simulink model "IEEE34_SPSload"  (R2021b)
settings: Solver=ode4  StartTime=0.0  StopTime=5  FixedStep=50e-6  RelTol=1e-3
PreLoadFcn:
  | pGain = 0.05; % Gain of random perturbation (pu)
  | pGainAP = 0.01; % Gain of sinusoidal active power variation (pu)
  | pGainRP = 0.01; % Gain of sinusoidal reactive power variation (pu)
  | pFreqAP = 0.03; % Frequency of sinusoidal active power variation (Hz)
  | pFreqRP = 0.03; % Frequency of sinusoidal reactive power variation (Hz)
  | 
  | init_IEEE34nodetestfeeder;
InitFcn:
  | pGain = 0.05; % Gain of random perturbation (pu)
  | pGainAP = 0.01; % Gain of sinusoidal active power variation (pu)
  | pGainRP = 0.01; % Gain of sinusoidal reactive power variation (pu)
  | pFreqAP = 0.03; % Frequency of sinusoidal active power variation (Hz)
  | pFreqRP = 0.03; % Frequency of sinusoidal reactive power variation (Hz)
  | 
  | init_IEEE34nodetestfeeder;
values from neighbouring files (symbols this model uses):
  fNom = f    (= 60)    [init_IEEE34nodetestfeeder.m]
  loadcoeff = 1.0    (= 1)    [init_IEEE34nodetestfeeder.m]
  Ts = 50e-6    (= 5e-05)    [init_IEEE34nodetestfeeder.m]
  vNomMV = VsubL    (= 24900)    [init_IEEE34nodetestfeeder.m]
  VsubL = 24.9e3    (= 24900)    [init_IEEE34nodetestfeeder.m]
  VxfmL = 4.16e3    (= 4160)    [init_IEEE34nodetestfeeder.m]
undefined symbols (not defined in the file or in its folder): Ac, Bc, Cc, Dc, find_system, j
libraries: spsSeriesRLCBranchLib x418, spsGroundLib x242, simulink_extras x176, spsVoltageMeasurementLib x106, spsRMSLib x96, spsControlledCurrentSourceLib x94, spsThreePhaseVIMeasurementLib x37, spsMutualInductanceLib x24, spsCurrentMeasurementLib x12, spsOnDelayLib x12, spsLinearTransformerLib x6, spsControlledVoltageSourceLib x6
(part 9 of 33)

== system IEEE34_SPSload/SM_IEEE34/DL_802-1/Load B ==
  Controlled Current Source : spsControlledCurrentSourceLib/Controlled Current Source  Initialize=on  Source_Type=AC  Amplitude=0  Phase=0  Frequency=0  Measurements=None
  Gain : Gain  Gain=-1
  Measurement list : Subsystem
  PQ : Ground
  Series RLC Branch : spsSeriesRLCBranchLib/Series RLC Branch  LConnTagsString=__new0  RConnTagsString=__new0  BranchType=R  Resistance=1e8  Inductance=1e-3  SetiL0=off  InitialCurrent=0  Capacitance=1e-6  Setx0=off  InitialVoltage=0  Measurements=None
  Voltage Measurement1 : spsVoltageMeasurementLib/Voltage Measurement  PhasorSimulation=off  OutputType=Complex  PSBequivalent=0
  model : Subsystem
  a : PMIOPort  Tag=PMCPort  Side=Left
  b : PMIOPort  Tag=PMCPort  Port=2  Side=Left
  m : Outport  InitialOutput=[0,0,0]  VectorParamsAs1DForOutWhenUnconnected=off
  wires:
  Gain/1 -> Controlled Current Source/1
  Measurement list/1(Out1) -> m/1
  model/1(i) -> Gain/1
  Voltage Measurement1/1 -> model/1(v)
  PQ/1 -> model/2(PQ)
  model/2(m) -> Measurement list/1(In1)
  connections:
  Series RLC Branch/RConn1 -- Voltage Measurement1/LConn2 -- b/RConn1 -- Controlled Current Source/LConn1
  a/RConn1 -- Series RLC Branch/LConn1 -- Controlled Current Source/RConn1 -- Voltage Measurement1/LConn1

== system IEEE34_SPSload/SM_IEEE34/DL_802-1/Load B1 ==
  Controlled Current Source : spsControlledCurrentSourceLib/Controlled Current Source  Initialize=on  Source_Type=AC  Amplitude=0  Phase=0  Frequency=0  Measurements=None
  Gain : Gain  Gain=-1
  Measurement list : Subsystem
  PQ : Ground
  Series RLC Branch : spsSeriesRLCBranchLib/Series RLC Branch  LConnTagsString=__new0  RConnTagsString=__new0  BranchType=R  Resistance=1e8  Inductance=1e-3  SetiL0=off  InitialCurrent=0  Capacitance=1e-6  Setx0=off  InitialVoltage=0  Measurements=None
  Voltage Measurement1 : spsVoltageMeasurementLib/Voltage Measurement  PhasorSimulation=off  OutputType=Complex  PSBequivalent=0
  model : Subsystem
  a : PMIOPort  Tag=PMCPort  Side=Left
  b : PMIOPort  Tag=PMCPort  Port=2  Side=Left
  m : Outport  InitialOutput=[0,0,0]  VectorParamsAs1DForOutWhenUnconnected=off
  wires:
  model/2(m) -> Measurement list/1(In1)
  PQ/1 -> model/2(PQ)
  Voltage Measurement1/1 -> model/1(v)
  model/1(i) -> Gain/1
  Measurement list/1(Out1) -> m/1
  Gain/1 -> Controlled Current Source/1
  connections:
  Voltage Measurement1/LConn1 -- Controlled Current Source/RConn1 -- Series RLC Branch/LConn1 -- a/RConn1
  Controlled Current Source/LConn1 -- b/RConn1 -- Voltage Measurement1/LConn2 -- Series RLC Branch/RConn1

== system IEEE34_SPSload/SM_IEEE34/DL_802-1/Load C ==
  Controlled Current Source : spsControlledCurrentSourceLib/Controlled Current Source  Initialize=on  Source_Type=AC  Amplitude=0  Phase=0  Frequency=0  Measurements=None
  Gain : Gain  Gain=-1
  Measurement list : Subsystem
  PQ : Ground
  Series RLC Branch : spsSeriesRLCBranchLib/Series RLC Branch  LConnTagsString=__new0  RConnTagsString=__new0  BranchType=R  Resistance=1e8  Inductance=1e-3  SetiL0=off  InitialCurrent=0  Capacitance=1e-6  Setx0=off  InitialVoltage=0  Measurements=None
  Voltage Measurement1 : spsVoltageMeasurementLib/Voltage Measurement  PhasorSimulation=off  OutputType=Complex  PSBequivalent=0
  model : Subsystem
  a : PMIOPort  Tag=PMCPort  Side=Left
  b : PMIOPort  Tag=PMCPort  Port=2  Side=Left
  m : Outport  InitialOutput=[0,0,0]  VectorParamsAs1DForOutWhenUnconnected=off
  wires:
  model/2(m) -> Measurement list/1(In1)
  PQ/1 -> model/2(PQ)
  Voltage Measurement1/1 -> model/1(v)
  model/1(i) -> Gain/1
  Measurement list/1(Out1) -> m/1
  Gain/1 -> Controlled Current Source/1
  connections:
  Voltage Measurement1/LConn1 -- a/RConn1 -- Series RLC Branch/LConn1 -- Controlled Current Source/RConn1
  Voltage Measurement1/LConn2 -- b/RConn1 -- Series RLC Branch/RConn1 -- Controlled Current Source/LConn1

== system IEEE34_SPSload/SM_IEEE34/DL_802-2/Load B ==
  Controlled Current Source : spsControlledCurrentSourceLib/Controlled Current Source  Initialize=on  Source_Type=AC  Amplitude=0  Phase=0  Frequency=0  Measurements=None
  Gain : Gain  Gain=-1
  Measurement list : Subsystem
  PQ : Ground
  Series RLC Branch : spsSeriesRLCBranchLib/Series RLC Branch  LConnTagsString=__new0  RConnTagsString=__new0  BranchType=R  Resistance=1e8  Inductance=1e-3  SetiL0=off  InitialCurrent=0  Capacitance=1e-6  Setx0=off  InitialVoltage=0  Measurements=None
  Voltage Measurement1 : spsVoltageMeasurementLib/Voltage Measurement  PhasorSimulation=off  OutputType=Complex  PSBequivalent=0
  model : Subsystem
  a : PMIOPort  Tag=PMCPort  Side=Left
  b : PMIOPort  Tag=PMCPort  Port=2  Side=Left
  m : Outport  InitialOutput=[0,0,0]  VectorParamsAs1DForOutWhenUnconnected=off
  wires:
  model/2(m) -> Measurement list/1(In1)
  PQ/1 -> model/2(PQ)
  Voltage Measurement1/1 -> model/1(v)
  model/1(i) -> Gain/1
  Measurement list/1(Out1) -> m/1
  Gain/1 -> Controlled Current Source/1
  connections:
  Voltage Measurement1/LConn1 -- Controlled Current Source/RConn1 -- Series RLC Branch/LConn1 -- a/RConn1
  Controlled Current Source/LConn1 -- b/RConn1 -- Voltage Measurement1/LConn2 -- Series RLC Branch/RConn1

== system IEEE34_SPSload/SM_IEEE34/DL_802-2/Load B1 ==
  Controlled Current Source : spsControlledCurrentSourceLib/Controlled Current Source  Initialize=on  Source_Type=AC  Amplitude=0  Phase=0  Frequency=0  Measurements=None
  Gain : Gain  Gain=-1
  Measurement list : Subsystem
  PQ : Ground
  Series RLC Branch : spsSeriesRLCBranchLib/Series RLC Branch  LConnTagsString=__new0  RConnTagsString=__new0  BranchType=R  Resistance=1e8  Inductance=1e-3  SetiL0=off  InitialCurrent=0  Capacitance=1e-6  Setx0=off  InitialVoltage=0  Measurements=None
  Voltage Measurement1 : spsVoltageMeasurementLib/Voltage Measurement  PhasorSimulation=off  OutputType=Complex  PSBequivalent=0
  model : Subsystem
  a : PMIOPort  Tag=PMCPort  Side=Left
  b : PMIOPort  Tag=PMCPort  Port=2  Side=Left
  m : Outport  InitialOutput=[0,0,0]  VectorParamsAs1DForOutWhenUnconnected=off
  wires:
  Gain/1 -> Controlled Current Source/1
  Measurement list/1(Out1) -> m/1
  model/1(i) -> Gain/1
  Voltage Measurement1/1 -> model/1(v)
  PQ/1 -> model/2(PQ)
  model/2(m) -> Measurement list/1(In1)
  connections:
  Series RLC Branch/RConn1 -- Voltage Measurement1/LConn2 -- b/RConn1 -- Controlled Current Source/LConn1
  a/RConn1 -- Series RLC Branch/LConn1 -- Controlled Current Source/RConn1 -- Voltage Measurement1/LConn1

== system IEEE34_SPSload/SM_IEEE34/DL_802-2/Load C ==
  Controlled Current Source : spsControlledCurrentSourceLib/Controlled Current Source  Initialize=on  Source_Type=AC  Amplitude=0  Phase=0  Frequency=0  Measurements=None
  Gain : Gain  Gain=-1
  Measurement list : Subsystem
  PQ : Ground
  Series RLC Branch : spsSeriesRLCBranchLib/Series RLC Branch  LConnTagsString=__new0  RConnTagsString=__new0  BranchType=R  Resistance=1e8  Inductance=1e-3  SetiL0=off  InitialCurrent=0  Capacitance=1e-6  Setx0=off  InitialVoltage=0  Measurements=None
  Voltage Measurement1 : spsVoltageMeasurementLib/Voltage Measurement  PhasorSimulation=off  OutputType=Complex  PSBequivalent=0
  model : Subsystem
  a : PMIOPort  Tag=PMCPort  Side=Left
  b : PMIOPort  Tag=PMCPort  Port=2  Side=Left
  m : Outport  InitialOutput=[0,0,0]  VectorParamsAs1DForOutWhenUnconnected=off
  wires:
  Gain/1 -> Controlled Current Source/1
  Measurement list/1(Out1) -> m/1
  model/1(i) -> Gain/1
  Voltage Measurement1/1 -> model/1(v)
  PQ/1 -> model/2(PQ)
  model/2(m) -> Measurement list/1(In1)
  connections:
  Controlled Current Source/LConn1 -- Series RLC Branch/RConn1 -- b/RConn1 -- Voltage Measurement1/LConn2
  Controlled Current Source/RConn1 -- Series RLC Branch/LConn1 -- a/RConn1 -- Voltage Measurement1/LConn1

== system IEEE34_SPSload/SM_IEEE34/DL_808-1/Load B ==
  Controlled Current Source : spsControlledCurrentSourceLib/Controlled Current Source  Initialize=on  Source_Type=AC  Amplitude=0  Phase=0  Frequency=0  Measurements=None
  Gain : Gain  Gain=-1
  Measurement list : Subsystem
  PQ : Ground
  Series RLC Branch : spsSeriesRLCBranchLib/Series RLC Branch  LConnTagsString=__new0  RConnTagsString=__new0  BranchType=R  Resistance=1e8  Inductance=1e-3  SetiL0=off  InitialCurrent=0  Capacitance=1e-6  Setx0=off  InitialVoltage=0  Measurements=None
  Voltage Measurement1 : spsVoltageMeasurementLib/Voltage Measurement  PhasorSimulation=off  OutputType=Complex  PSBequivalent=0
  model : Subsystem
  a : PMIOPort  Tag=PMCPort  Side=Left
  b : PMIOPort  Tag=PMCPort  Port=2  Side=Left
  m : Outport  InitialOutput=[0,0,0]  VectorParamsAs1DForOutWhenUnconnected=off
  wires:
  Gain/1 -> Controlled Current Source/1
  Measurement list/1(Out1) -> m/1
  model/1(i) -> Gain/1
  Voltage Measurement1/1 -> model/1(v)
  PQ/1 -> model/2(PQ)
  model/2(m) -> Measurement list/1(In1)
  connections:
  Controlled Current Source/LConn1 -- b/RConn1 -- Series RLC Branch/RConn1 -- Voltage Measurement1/LConn2
  Controlled Current Source/RConn1 -- a/RConn1 -- Series RLC Branch/LConn1 -- Voltage Measurement1/LConn1

== system IEEE34_SPSload/SM_IEEE34/DL_808-810/Load B ==
  Controlled Current Source : spsControlledCurrentSourceLib/Controlled Current Source  Initialize=on  Source_Type=AC  Amplitude=0  Phase=0  Frequency=0  Measurements=None
  Gain : Gain  Gain=-1
  Measurement list : Subsystem
  PQ : Ground
  Series RLC Branch : spsSeriesRLCBranchLib/Series RLC Branch  LConnTagsString=__new0  RConnTagsString=__new0  BranchType=R  Resistance=1e8  Inductance=1e-3  SetiL0=off  InitialCurrent=0  Capacitance=1e-6  Setx0=off  InitialVoltage=0  Measurements=None
  Voltage Measurement1 : spsVoltageMeasurementLib/Voltage Measurement  PhasorSimulation=off  OutputType=Complex  PSBequivalent=0
  model : Subsystem
  a : PMIOPort  Tag=PMCPort  Side=Left
  b : PMIOPort  Tag=PMCPort  Port=2  Side=Left
  m : Outport  InitialOutput=[0,0,0]  VectorParamsAs1DForOutWhenUnconnected=off
  wires:
  model/2(m) -> Measurement list/1(In1)
  PQ/1 -> model/2(PQ)
  Voltage Measurement1/1 -> model/1(v)
  model/1(i) -> Gain/1
  Measurement list/1(Out1) -> m/1
  Gain/1 -> Controlled Current Source/1
  connections:
  Voltage Measurement1/LConn1 -- Series RLC Branch/LConn1 -- a/RConn1 -- Controlled Current Source/RConn1
  Voltage Measurement1/LConn2 -- Series RLC Branch/RConn1 -- b/RConn1 -- Controlled Current Source/LConn1

== system IEEE34_SPSload/SM_IEEE34/DL_816-1/Load B ==
  Controlled Current Source : spsControlledCurrentSourceLib/Controlled Current Source  Initialize=on  Source_Type=AC  Amplitude=0  Phase=0  Frequency=0  Measurements=None
  Gain : Gain  Gain=-1
  Measurement list : Subsystem
  PQ : Ground
  Series RLC Branch : spsSeriesRLCBranchLib/Series RLC Branch  LConnTagsString=__new0  RConnTagsString=__new0  BranchType=R  Resistance=1e8  Inductance=1e-3  SetiL0=off  InitialCurrent=0  Capacitance=1e-6  Setx0=off  InitialVoltage=0  Measurements=None
  Voltage Measurement1 : spsVoltageMeasurementLib/Voltage Measurement  PhasorSimulation=off  OutputType=Complex  PSBequivalent=0
  model : Subsystem
  a : PMIOPort  Tag=PMCPort  Side=Left
  b : PMIOPort  Tag=PMCPort  Port=2  Side=Left
  m : Outport  InitialOutput=[0,0,0]  VectorParamsAs1DForOutWhenUnconnected=off
  wires:
  Gain/1 -> Controlled Current Source/1
  Measurement list/1(Out1) -> m/1
  model/1(i) -> Gain/1
  Voltage Measurement1/1 -> model/1(v)
  PQ/1 -> model/2(PQ)
  model/2(m) -> Measurement list/1(In1)
  connections:
  Controlled Current Source/LConn1 -- b/RConn1 -- Series RLC Branch/RConn1 -- Voltage Measurement1/LConn2
  Controlled Current Source/RConn1 -- a/RConn1 -- Series RLC Branch/LConn1 -- Voltage Measurement1/LConn1

== system IEEE34_SPSload/SM_IEEE34/DL_816-1/Load B1 ==
  Controlled Current Source : spsControlledCurrentSourceLib/Controlled Current Source  Initialize=on  Source_Type=AC  Amplitude=0  Phase=0  Frequency=0  Measurements=None
  Gain : Gain  Gain=-1
  Measurement list : Subsystem
  PQ : Ground
  Series RLC Branch : spsSeriesRLCBranchLib/Series RLC Branch  LConnTagsString=__new0  RConnTagsString=__new0  BranchType=R  Resistance=1e8  Inductance=1e-3  SetiL0=off  InitialCurrent=0  Capacitance=1e-6  Setx0=off  InitialVoltage=0  Measurements=None
  Voltage Measurement1 : spsVoltageMeasurementLib/Voltage Measurement  PhasorSimulation=off  OutputType=Complex  PSBequivalent=0
  model : Subsystem
  a : PMIOPort  Tag=PMCPort  Side=Left
  b : PMIOPort  Tag=PMCPort  Port=2  Side=Left
  m : Outport  InitialOutput=[0,0,0]  VectorParamsAs1DForOutWhenUnconnected=off
  wires:
  model/2(m) -> Measurement list/1(In1)
  PQ/1 -> model/2(PQ)
  Voltage Measurement1/1 -> model/1(v)
  model/1(i) -> Gain/1
  Measurement list/1(Out1) -> m/1
  Gain/1 -> Controlled Current Source/1
  connections:
  Voltage Measurement1/LConn1 -- Series RLC Branch/LConn1 -- a/RConn1 -- Controlled Current Source/RConn1
  Voltage Measurement1/LConn2 -- Series RLC Branch/RConn1 -- b/RConn1 -- Controlled Current Source/LConn1

== system IEEE34_SPSload/SM_IEEE34/DL_816-1/Load B2 ==
  Controlled Current Source : spsControlledCurrentSourceLib/Controlled Current Source  Initialize=on  Source_Type=AC  Amplitude=0  Phase=0  Frequency=0  Measurements=None
  Gain : Gain  Gain=-1
  Measurement list : Subsystem
  PQ : Ground
  Series RLC Branch : spsSeriesRLCBranchLib/Series RLC Branch  LConnTagsString=__new0  RConnTagsString=__new0  BranchType=R  Resistance=1e8  Inductance=1e-3  SetiL0=off  InitialCurrent=0  Capacitance=1e-6  Setx0=off  InitialVoltage=0  Measurements=None
  Voltage Measurement1 : spsVoltageMeasurementLib/Voltage Measurement  PhasorSimulation=off  OutputType=Complex  PSBequivalent=0
  model : Subsystem
  a : PMIOPort  Tag=PMCPort  Side=Left
  b : PMIOPort  Tag=PMCPort  Port=2  Side=Left
  m : Outport  InitialOutput=[0,0,0]  VectorParamsAs1DForOutWhenUnconnected=off
  wires:
  model/2(m) -> Measurement list/1(In1)
  PQ/1 -> model/2(PQ)
  Voltage Measurement1/1 -> model/1(v)
  model/1(i) -> Gain/1
  Measurement list/1(Out1) -> m/1
  Gain/1 -> Controlled Current Source/1
  connections:
  Voltage Measurement1/LConn1 -- Series RLC Branch/LConn1 -- a/RConn1 -- Controlled Current Source/RConn1
  Voltage Measurement1/LConn2 -- Series RLC Branch/RConn1 -- b/RConn1 -- Controlled Current Source/LConn1

== system IEEE34_SPSload/SM_IEEE34/DL_816-824/Load B ==
  Controlled Current Source : spsControlledCurrentSourceLib/Controlled Current Source  Initialize=on  Source_Type=AC  Amplitude=0  Phase=0  Frequency=0  Measurements=None
  Gain : Gain  Gain=-1
  Measurement list : Subsystem
  PQ : Ground
  Series RLC Branch : spsSeriesRLCBranchLib/Series RLC Branch  LConnTagsString=__new0  RConnTagsString=__new0  BranchType=R  Resistance=1e8  Inductance=1e-3  SetiL0=off  InitialCurrent=0  Capacitance=1e-6  Setx0=off  InitialVoltage=0  Measurements=None
  Voltage Measurement1 : spsVoltageMeasurementLib/Voltage Measurement  PhasorSimulation=off  OutputType=Complex  PSBequivalent=0
  model : Subsystem
  a : PMIOPort  Tag=PMCPort  Side=Left
  b : PMIOPort  Tag=PMCPort  Port=2  Side=Left
  m : Outport  InitialOutput=[0,0,0]  VectorParamsAs1DForOutWhenUnconnected=off
  wires:
  model/2(m) -> Measurement list/1(In1)
  PQ/1 -> model/2(PQ)
  Voltage Measurement1/1 -> model/1(v)
  model/1(i) -> Gain/1
  Measurement list/1(Out1) -> m/1
  Gain/1 -> Controlled Current Source/1
  connections:
  Voltage Measurement1/LConn1 -- Series RLC Branch/LConn1 -- a/RConn1 -- Controlled Current Source/RConn1
  Voltage Measurement1/LConn2 -- Series RLC Branch/RConn1 -- b/RConn1 -- Controlled Current Source/LConn1

== system IEEE34_SPSload/SM_IEEE34/DL_816-824/Load B1 ==
  Controlled Current Source : spsControlledCurrentSourceLib/Controlled Current Source  Initialize=on  Source_Type=AC  Amplitude=0  Phase=0  Frequency=0  Measurements=None
  Gain : Gain  Gain=-1
  Measurement list : Subsystem
  PQ : Ground
  Series RLC Branch : spsSeriesRLCBranchLib/Series RLC Branch  LConnTagsString=__new0  RConnTagsString=__new0  BranchType=R  Resistance=1e8  Inductance=1e-3  SetiL0=off  InitialCurrent=0  Capacitance=1e-6  Setx0=off  InitialVoltage=0  Measurements=None
  Voltage Measurement1 : spsVoltageMeasurementLib/Voltage Measurement  PhasorSimulation=off  OutputType=Complex  PSBequivalent=0
  model : Subsystem
  a : PMIOPort  Tag=PMCPort  Side=Left
  b : PMIOPort  Tag=PMCPort  Port=2  Side=Left
  m : Outport  InitialOutput=[0,0,0]  VectorParamsAs1DForOutWhenUnconnected=off
  wires:
  Gain/1 -> Controlled Current Source/1
  Measurement list/1(Out1) -> m/1
  model/1(i) -> Gain/1
  Voltage Measurement1/1 -> model/1(v)
  PQ/1 -> model/2(PQ)
  model/2(m) -> Measurement list/1(In1)
  connections:
  Controlled Current Source/LConn1 -- b/RConn1 -- Series RLC Branch/RConn1 -- Voltage Measurement1/LConn2
  Controlled Current Source/RConn1 -- a/RConn1 -- Series RLC Branch/LConn1 -- Voltage Measurement1/LConn1

== system IEEE34_SPSload/SM_IEEE34/DL_816-824/Load B2 ==
  Controlled Current Source : spsControlledCurrentSourceLib/Controlled Current Source  Initialize=on  Source_Type=AC  Amplitude=0  Phase=0  Frequency=0  Measurements=None
  Gain : Gain  Gain=-1
  Measurement list : Subsystem
  PQ : Ground
  Series RLC Branch : spsSeriesRLCBranchLib/Series RLC Branch  LConnTagsString=__new0  RConnTagsString=__new0  BranchType=R  Resistance=1e8  Inductance=1e-3  SetiL0=off  InitialCurrent=0  Capacitance=1e-6  Setx0=off  InitialVoltage=0  Measurements=None
  Voltage Measurement1 : spsVoltageMeasurementLib/Voltage Measurement  PhasorSimulation=off  OutputType=Complex  PSBequivalent=0
  model : Subsystem
  a : PMIOPort  Tag=PMCPort  Side=Left
  b : PMIOPort  Tag=PMCPort  Port=2  Side=Left
  m : Outport  InitialOutput=[0,0,0]  VectorParamsAs1DForOutWhenUnconnected=off
  wires:
  Gain/1 -> Controlled Current Source/1
  Measurement list/1(Out1) -> m/1
  model/1(i) -> Gain/1
  Voltage Measurement1/1 -> model/1(v)
  PQ/1 -> model/2(PQ)
  model/2(m) -> Measurement list/1(In1)
  connections:
  Controlled Current Source/LConn1 -- b/RConn1 -- Series RLC Branch/RConn1 -- Voltage Measurement1/LConn2
  Controlled Current Source/RConn1 -- a/RConn1 -- Series RLC Branch/LConn1 -- Voltage Measurement1/LConn1

== system IEEE34_SPSload/SM_IEEE34/DL_818-1/Load B ==
  Controlled Current Source : spsControlledCurrentSourceLib/Controlled Current Source  Initialize=on  Source_Type=AC  Amplitude=0  Phase=0  Frequency=0  Measurements=None
  Gain : Gain  Gain=-1
  Measurement list : Subsystem
  PQ : Ground
  Series RLC Branch : spsSeriesRLCBranchLib/Series RLC Branch  LConnTagsString=__new0  RConnTagsString=__new0  BranchType=R  Resistance=1e8  Inductance=1e-3  SetiL0=off  InitialCurrent=0  Capacitance=1e-6  Setx0=off  InitialVoltage=0  Measurements=None
  Voltage Measurement1 : spsVoltageMeasurementLib/Voltage Measurement  PhasorSimulation=off  OutputType=Complex  PSBequivalent=0
  model : Subsystem
  a : PMIOPort  Tag=PMCPort  Side=Left
  b : PMIOPort  Tag=PMCPort  Port=2  Side=Left
  m : Outport  InitialOutput=[0,0,0]  VectorParamsAs1DForOutWhenUnconnected=off
  wires:
  Gain/1 -> Controlled Current Source/1
  Measurement list/1(Out1) -> m/1
  model/1(i) -> Gain/1
  Voltage Measurement1/1 -> model/1(v)
  PQ/1 -> model/2(PQ)
  model/2(m) -> Measurement list/1(In1)
  connections:
  Controlled Current Source/LConn1 -- b/RConn1 -- Series RLC Branch/RConn1 -- Voltage Measurement1/LConn2
  Controlled Current Source/RConn1 -- a/RConn1 -- Series RLC Branch/LConn1 -- Voltage Measurement1/LConn1

== system IEEE34_SPSload/SM_IEEE34/DL_818-820/Load B ==
  Controlled Current Source : spsControlledCurrentSourceLib/Controlled Current Source  Initialize=on  Source_Type=AC  Amplitude=0  Phase=0  Frequency=0  Measurements=None
  Gain : Gain  Gain=-1
  Measurement list : Subsystem
  PQ : Ground
  Series RLC Branch : spsSeriesRLCBranchLib/Series RLC Branch  LConnTagsString=__new0  RConnTagsString=__new0  BranchType=R  Resistance=1e8  Inductance=1e-3  SetiL0=off  InitialCurrent=0  Capacitance=1e-6  Setx0=off  InitialVoltage=0  Measurements=None
  Voltage Measurement1 : spsVoltageMeasurementLib/Voltage Measurement  PhasorSimulation=off  OutputType=Complex  PSBequivalent=0
  model : Subsystem
  a : PMIOPort  Tag=PMCPort  Side=Left
  b : PMIOPort  Tag=PMCPort  Port=2  Side=Left
  m : Outport  InitialOutput=[0,0,0]  VectorParamsAs1DForOutWhenUnconnected=off
  wires:
  model/2(m) -> Measurement list/1(In1)
  PQ/1 -> model/2(PQ)
  Voltage Measurement1/1 -> model/1(v)
  model/1(i) -> Gain/1
  Measurement list/1(Out1) -> m/1
  Gain/1 -> Controlled Current Source/1
  connections:
  Voltage Measurement1/LConn1 -- Series RLC Branch/LConn1 -- a/RConn1 -- Controlled Current Source/RConn1
  Voltage Measurement1/LConn2 -- Series RLC Branch/RConn1 -- b/RConn1 -- Controlled Current Source/LConn1

== system IEEE34_SPSload/SM_IEEE34/DL_820-1/Load B ==
  Controlled Current Source : spsControlledCurrentSourceLib/Controlled Current Source  Initialize=on  Source_Type=AC  Amplitude=0  Phase=0  Frequency=0  Measurements=None
  Gain : Gain  Gain=-1
  Measurement list : Subsystem
  PQ : Ground
  Series RLC Branch : spsSeriesRLCBranchLib/Series RLC Branch  LConnTagsString=__new0  RConnTagsString=__new0  BranchType=R  Resistance=1e8  Inductance=1e-3  SetiL0=off  InitialCurrent=0  Capacitance=1e-6  Setx0=off  InitialVoltage=0  Measurements=None
  Voltage Measurement1 : spsVoltageMeasurementLib/Voltage Measurement  PhasorSimulation=off  OutputType=Complex  PSBequivalent=0
  model : Subsystem
  a : PMIOPort  Tag=PMCPort  Side=Left
  b : PMIOPort  Tag=PMCPort  Port=2  Side=Left
  m : Outport  InitialOutput=[0,0,0]  VectorParamsAs1DForOutWhenUnconnected=off
  wires:
  Gain/1 -> Controlled Current Source/1
  Measurement list/1(Out1) -> m/1
  model/1(i) -> Gain/1
  Voltage Measurement1/1 -> model/1(v)
  PQ/1 -> model/2(PQ)
  model/2(m) -> Measurement list/1(In1)
  connections:
  Controlled Current Source/LConn1 -- b/RConn1 -- Series RLC Branch/RConn1 -- Voltage Measurement1/LConn2
  Controlled Current Source/RConn1 -- a/RConn1 -- Series RLC Branch/LConn1 -- Voltage Measurement1/LConn1

== system IEEE34_SPSload/SM_IEEE34/DL_820-822/Load B ==
  Controlled Current Source : spsControlledCurrentSourceLib/Controlled Current Source  Initialize=on  Source_Type=AC  Amplitude=0  Phase=0  Frequency=0  Measurements=None
  Gain : Gain  Gain=-1
  Measurement list : Subsystem
  PQ : Ground
  Series RLC Branch : spsSeriesRLCBranchLib/Series RLC Branch  LConnTagsString=__new0  RConnTagsString=__new0  BranchType=R  Resistance=1e8  Inductance=1e-3  SetiL0=off  InitialCurrent=0  Capacitance=1e-6  Setx0=off  InitialVoltage=0  Measurements=None
  Voltage Measurement1 : spsVoltageMeasurementLib/Voltage Measurement  PhasorSimulation=off  OutputType=Complex  PSBequivalent=0
  model : Subsystem
  a : PMIOPort  Tag=PMCPort  Side=Left
  b : PMIOPort  Tag=PMCPort  Port=2  Side=Left
  m : Outport  InitialOutput=[0,0,0]  VectorParamsAs1DForOutWhenUnconnected=off
  wires:
  model/2(m) -> Measurement list/1(In1)
  PQ/1 -> model/2(PQ)
  Voltage Measurement1/1 -> model/1(v)
  model/1(i) -> Gain/1
  Measurement list/1(Out1) -> m/1
  Gain/1 -> Controlled Current Source/1
  connections:
  Voltage Measurement1/LConn1 -- Series RLC Branch/LConn1 -- a/RConn1 -- Controlled Current Source/RConn1
  Voltage Measurement1/LConn2 -- Series RLC Branch/RConn1 -- b/RConn1 -- Controlled Current Source/LConn1

== system IEEE34_SPSload/SM_IEEE34/DL_824-1/Load B ==
  Controlled Current Source : spsControlledCurrentSourceLib/Controlled Current Source  Initialize=on  Source_Type=AC  Amplitude=0  Phase=0  Frequency=0  Measurements=None
  Gain : Gain  Gain=-1
  Measurement list : Subsystem
  PQ : Ground
  Series RLC Branch : spsSeriesRLCBranchLib/Series RLC Branch  LConnTagsString=__new0  RConnTagsString=__new0  BranchType=R  Resistance=1e8  Inductance=1e-3  SetiL0=off  InitialCurrent=0  Capacitance=1e-6  Setx0=off  InitialVoltage=0  Measurements=None
  Voltage Measurement1 : spsVoltageMeasurementLib/Voltage Measurement  PhasorSimulation=off  OutputType=Complex  PSBequivalent=0
  model : Subsystem
  a : PMIOPort  Tag=PMCPort  Side=Left
  b : PMIOPort  Tag=PMCPort  Port=2  Side=Left
  m : Outport  InitialOutput=[0,0,0]  VectorParamsAs1DForOutWhenUnconnected=off
  wires:
  model/2(m) -> Measurement list/1(In1)
  PQ/1 -> model/2(PQ)
  Voltage Measurement1/1 -> model/1(v)
  model/1(i) -> Gain/1
  Measurement list/1(Out1) -> m/1
  Gain/1 -> Controlled Current Source/1
  connections:
  Voltage Measurement1/LConn1 -- Series RLC Branch/LConn1 -- a/RConn1 -- Controlled Current Source/RConn1
  Voltage Measurement1/LConn2 -- Series RLC Branch/RConn1 -- b/RConn1 -- Controlled Current Source/LConn1

== system IEEE34_SPSload/SM_IEEE34/DL_824-2/Load B ==
  Controlled Current Source : spsControlledCurrentSourceLib/Controlled Current Source  Initialize=on  Source_Type=AC  Amplitude=0  Phase=0  Frequency=0  Measurements=None
  Gain : Gain  Gain=-1
  Measurement list : Subsystem
  PQ : Ground
  Series RLC Branch : spsSeriesRLCBranchLib/Series RLC Branch  LConnTagsString=__new0  RConnTagsString=__new0  BranchType=R  Resistance=1e8  Inductance=1e-3  SetiL0=off  InitialCurrent=0  Capacitance=1e-6  Setx0=off  InitialVoltage=0  Measurements=None
  Voltage Measurement1 : spsVoltageMeasurementLib/Voltage Measurement  PhasorSimulation=off  OutputType=Complex  PSBequivalent=0
  model : Subsystem
  a : PMIOPort  Tag=PMCPort  Side=Left
  b : PMIOPort  Tag=PMCPort  Port=2  Side=Left
  m : Outport  InitialOutput=[0,0,0]  VectorParamsAs1DForOutWhenUnconnected=off
  wires:
  Gain/1 -> Controlled Current Source/1
  Measurement list/1(Out1) -> m/1
  model/1(i) -> Gain/1
  Voltage Measurement1/1 -> model/1(v)
  PQ/1 -> model/2(PQ)
  model/2(m) -> Measurement list/1(In1)
  connections:
  Controlled Current Source/LConn1 -- b/RConn1 -- Series RLC Branch/RConn1 -- Voltage Measurement1/LConn2
  Controlled Current Source/RConn1 -- a/RConn1 -- Series RLC Branch/LConn1 -- Voltage Measurement1/LConn1

== system IEEE34_SPSload/SM_IEEE34/DL_824-826/Load B ==
  Controlled Current Source : spsControlledCurrentSourceLib/Controlled Current Source  Initialize=on  Source_Type=AC  Amplitude=0  Phase=0  Frequency=0  Measurements=None
  Gain : Gain  Gain=-1
  Measurement list : Subsystem
  PQ : Ground
  Series RLC Branch : spsSeriesRLCBranchLib/Series RLC Branch  LConnTagsString=__new0  RConnTagsString=__new0  BranchType=R  Resistance=1e8  Inductance=1e-3  SetiL0=off  InitialCurrent=0  Capacitance=1e-6  Setx0=off  InitialVoltage=0  Measurements=None
  Voltage Measurement1 : spsVoltageMeasurementLib/Voltage Measurement  PhasorSimulation=off  OutputType=Complex  PSBequivalent=0
  model : Subsystem
  a : PMIOPort  Tag=PMCPort  Side=Left
  b : PMIOPort  Tag=PMCPort  Port=2  Side=Left
  m : Outport  InitialOutput=[0,0,0]  VectorParamsAs1DForOutWhenUnconnected=off
  wires:
  model/2(m) -> Measurement list/1(In1)
  PQ/1 -> model/2(PQ)
  Voltage Measurement1/1 -> model/1(v)
  model/1(i) -> Gain/1
  Measurement list/1(Out1) -> m/1
  Gain/1 -> Controlled Current Source/1
  connections:
  Voltage Measurement1/LConn1 -- Series RLC Branch/LConn1 -- a/RConn1 -- Controlled Current Source/RConn1
  Voltage Measurement1/LConn2 -- Series RLC Branch/RConn1 -- b/RConn1 -- Controlled Current Source/LConn1

== system IEEE34_SPSload/SM_IEEE34/DL_824-828/Load B ==
  Controlled Current Source : spsControlledCurrentSourceLib/Controlled Current Source  Initialize=on  Source_Type=AC  Amplitude=0  Phase=0  Frequency=0  Measurements=None
  Gain : Gain  Gain=-1
  Measurement list : Subsystem
  PQ : Ground
  Series RLC Branch : spsSeriesRLCBranchLib/Series RLC Branch  LConnTagsString=__new0  RConnTagsString=__new0  BranchType=R  Resistance=1e8  Inductance=1e-3  SetiL0=off  InitialCurrent=0  Capacitance=1e-6  Setx0=off  InitialVoltage=0  Measurements=None
  Voltage Measurement1 : spsVoltageMeasurementLib/Voltage Measurement  PhasorSimulation=off  OutputType=Complex  PSBequivalent=0
  model : Subsystem
  a : PMIOPort  Tag=PMCPort  Side=Left
  b : PMIOPort  Tag=PMCPort  Port=2  Side=Left
  m : Outport  InitialOutput=[0,0,0]  VectorParamsAs1DForOutWhenUnconnected=off
  wires:
  model/2(m) -> Measurement list/1(In1)
  PQ/1 -> model/2(PQ)
  Voltage Measurement1/1 -> model/1(v)
  model/1(i) -> Gain/1
  Measurement list/1(Out1) -> m/1
  Gain/1 -> Controlled Current Source/1
  connections:
  Voltage Measurement1/LConn1 -- Series RLC Branch/LConn1 -- a/RConn1 -- Controlled Current Source/RConn1
  Voltage Measurement1/LConn2 -- Series RLC Branch/RConn1 -- b/RConn1 -- Controlled Current Source/LConn1

== system IEEE34_SPSload/SM_IEEE34/DL_828-1/Load B ==
  Controlled Current Source : spsControlledCurrentSourceLib/Controlled Current Source  Initialize=on  Source_Type=AC  Amplitude=0  Phase=0  Frequency=0  Measurements=None
  Gain : Gain  Gain=-1
  Measurement list : Subsystem
  PQ : Ground
  Series RLC Branch : spsSeriesRLCBranchLib/Series RLC Branch  LConnTagsString=__new0  RConnTagsString=__new0  BranchType=R  Resistance=1e8  Inductance=1e-3  SetiL0=off  InitialCurrent=0  Capacitance=1e-6  Setx0=off  InitialVoltage=0  Measurements=None
  Voltage Measurement1 : spsVoltageMeasurementLib/Voltage Measurement  PhasorSimulation=off  OutputType=Complex  PSBequivalent=0
  model : Subsystem
  a : PMIOPort  Tag=PMCPort  Side=Left
  b : PMIOPort  Tag=PMCPort  Port=2  Side=Left
  m : Outport  InitialOutput=[0,0,0]  VectorParamsAs1DForOutWhenUnconnected=off
  wires:
  Gain/1 -> Controlled Current Source/1
  Measurement list/1(Out1) -> m/1
  model/1(i) -> Gain/1
  Voltage Measurement1/1 -> model/1(v)
  PQ/1 -> model/2(PQ)
  model/2(m) -> Measurement list/1(In1)
  connections:
  Controlled Current Source/LConn1 -- b/RConn1 -- Series RLC Branch/RConn1 -- Voltage Measurement1/LConn2
  Controlled Current Source/RConn1 -- a/RConn1 -- Series RLC Branch/LConn1 -- Voltage Measurement1/LConn1

== system IEEE34_SPSload/SM_IEEE34/DL_828-830/Load B ==
  Controlled Current Source : spsControlledCurrentSourceLib/Controlled Current Source  Initialize=on  Source_Type=AC  Amplitude=0  Phase=0  Frequency=0  Measurements=None
  Gain : Gain  Gain=-1
  Measurement list : Subsystem
  PQ : Ground
  Series RLC Branch : spsSeriesRLCBranchLib/Series RLC Branch  LConnTagsString=__new0  RConnTagsString=__new0  BranchType=R  Resistance=1e8  Inductance=1e-3  SetiL0=off  InitialCurrent=0  Capacitance=1e-6  Setx0=off  InitialVoltage=0  Measurements=None
  Voltage Measurement1 : spsVoltageMeasurementLib/Voltage Measurement  PhasorSimulation=off  OutputType=Complex  PSBequivalent=0
  model : Subsystem
  a : PMIOPort  Tag=PMCPort  Side=Left
  b : PMIOPort  Tag=PMCPort  Port=2  Side=Left
  m : Outport  InitialOutput=[0,0,0]  VectorParamsAs1DForOutWhenUnconnected=off
  wires:
  model/2(m) -> Measurement list/1(In1)
  PQ/1 -> model/2(PQ)
  Voltage Measurement1/1 -> model/1(v)
  model/1(i) -> Gain/1
  Measurement list/1(Out1) -> m/1
  Gain/1 -> Controlled Current Source/1
  connections:
  Voltage Measurement1/LConn1 -- Series RLC Branch/LConn1 -- a/RConn1 -- Controlled Current Source/RConn1
  Voltage Measurement1/LConn2 -- Series RLC Branch/RConn1 -- b/RConn1 -- Controlled Current Source/LConn1

== system IEEE34_SPSload/SM_IEEE34/DL_832-1/Load A ==
  Controlled Current Source : spsControlledCurrentSourceLib/Controlled Current Source  Initialize=on  Source_Type=AC  Amplitude=0  Phase=0  Frequency=0  Measurements=None
  Gain : Gain  Gain=-1
  Measurement list : Subsystem
  PQ : Ground
  Series RLC Branch : spsSeriesRLCBranchLib/Series RLC Branch  LConnTagsString=__new0  RConnTagsString=__new0  BranchType=R  Resistance=1e8  Inductance=1e-3  SetiL0=off  InitialCurrent=0  Capacitance=1e-6  Setx0=off  InitialVoltage=0  Measurements=None
  Voltage Measurement1 : spsVoltageMeasurementLib/Voltage Measurement  PhasorSimulation=off  OutputType=Complex  PSBequivalent=0
  model : Subsystem
  a : PMIOPort  Tag=PMCPort  Side=Left
  b : PMIOPort  Tag=PMCPort  Port=2  Side=Left
  m : Outport  InitialOutput=[0,0,0]  VectorParamsAs1DForOutWhenUnconnected=off
  wires:
  Gain/1 -> Controlled Current Source/1
  Measurement list/1(Out1) -> m/1
  model/1(i) -> Gain/1
  Voltage Measurement1/1 -> model/1(v)
  PQ/1 -> model/2(PQ)
  model/2(m) -> Measurement list/1(In1)
  connections:
  Controlled Current Source/LConn1 -- b/RConn1 -- Series RLC Branch/RConn1 -- Voltage Measurement1/LConn2
  Controlled Current Source/RConn1 -- a/RConn1 -- Series RLC Branch/LConn1 -- Voltage Measurement1/LConn1

== system IEEE34_SPSload/SM_IEEE34/DL_832-1/Load B ==
  Controlled Current Source : spsControlledCurrentSourceLib/Controlled Current Source  Initialize=on  Source_Type=AC  Amplitude=0  Phase=0  Frequency=0  Measurements=None
  Gain : Gain  Gain=-1
  Measurement list : Subsystem
  PQ : Ground
  Series RLC Branch : spsSeriesRLCBranchLib/Series RLC Branch  LConnTagsString=__new0  RConnTagsString=__new0  BranchType=R  Resistance=1e8  Inductance=1e-3  SetiL0=off  InitialCurrent=0  Capacitance=1e-6  Setx0=off  InitialVoltage=0  Measurements=None
  Voltage Measurement1 : spsVoltageMeasurementLib/Voltage Measurement  PhasorSimulation=off  OutputType=Complex  PSBequivalent=0
  model : Subsystem
  a : PMIOPort  Tag=PMCPort  Side=Left
  b : PMIOPort  Tag=PMCPort  Port=2  Side=Left
  m : Outport  InitialOutput=[0,0,0]  VectorParamsAs1DForOutWhenUnconnected=off
  wires:
  model/2(m) -> Measurement list/1(In1)
  PQ/1 -> model/2(PQ)
  Voltage Measurement1/1 -> model/1(v)
  model/1(i) -> Gain/1
  Measurement list/1(Out1) -> m/1
  Gain/1 -> Controlled Current Source/1
  connections:
  Voltage Measurement1/LConn1 -- Series RLC Branch/LConn1 -- a/RConn1 -- Controlled Current Source/RConn1
  Voltage Measurement1/LConn2 -- Series RLC Branch/RConn1 -- b/RConn1 -- Controlled Current Source/LConn1

== system IEEE34_SPSload/SM_IEEE34/DL_832-1/Load C ==
  Controlled Current Source : spsControlledCurrentSourceLib/Controlled Current Source  Initialize=on  Source_Type=AC  Amplitude=0  Phase=0  Frequency=0  Measurements=None
  Gain : Gain  Gain=-1
  Measurement list : Subsystem
  PQ : Ground
  Series RLC Branch : spsSeriesRLCBranchLib/Series RLC Branch  LConnTagsString=__new0  RConnTagsString=__new0  BranchType=R  Resistance=1e8  Inductance=1e-3  SetiL0=off  InitialCurrent=0  Capacitance=1e-6  Setx0=off  InitialVoltage=0  Measurements=None
  Voltage Measurement1 : spsVoltageMeasurementLib/Voltage Measurement  PhasorSimulation=off  OutputType=Complex  PSBequivalent=0
  model : Subsystem
  a : PMIOPort  Tag=PMCPort  Side=Left
  b : PMIOPort  Tag=PMCPort  Port=2  Side=Left
  m : Outport  InitialOutput=[0,0,0]  VectorParamsAs1DForOutWhenUnconnected=off
  wires:
  Gain/1 -> Controlled Current Source/1
  Measurement list/1(Out1) -> m/1
  model/1(i) -> Gain/1
  Voltage Measurement1/1 -> model/1(v)
  PQ/1 -> model/2(PQ)
  model/2(m) -> Measurement list/1(In1)
  connections:
  Controlled Current Source/LConn1 -- b/RConn1 -- Series RLC Branch/RConn1 -- Voltage Measurement1/LConn2
  Controlled Current Source/RConn1 -- a/RConn1 -- Series RLC Branch/LConn1 -- Voltage Measurement1/LConn1

== system IEEE34_SPSload/SM_IEEE34/DL_832-858/Load A ==
  Controlled Current Source : spsControlledCurrentSourceLib/Controlled Current Source  Initialize=on  Source_Type=AC  Amplitude=0  Phase=0  Frequency=0  Measurements=None
  Gain : Gain  Gain=-1
  Measurement list : Subsystem
  PQ : Ground
  Series RLC Branch : spsSeriesRLCBranchLib/Series RLC Branch  LConnTagsString=__new0  RConnTagsString=__new0  BranchType=R  Resistance=1e8  Inductance=1e-3  SetiL0=off  InitialCurrent=0  Capacitance=1e-6  Setx0=off  InitialVoltage=0  Measurements=None
  Voltage Measurement1 : spsVoltageMeasurementLib/Voltage Measurement  PhasorSimulation=off  OutputType=Complex  PSBequivalent=0
  model : Subsystem
  a : PMIOPort  Tag=PMCPort  Side=Left
  b : PMIOPort  Tag=PMCPort  Port=2  Side=Left
  m : Outport  InitialOutput=[0,0,0]  VectorParamsAs1DForOutWhenUnconnected=off
  wires:
  model/2(m) -> Measurement list/1(In1)
  PQ/1 -> model/2(PQ)
  Voltage Measurement1/1 -> model/1(v)
  model/1(i) -> Gain/1
  Measurement list/1(Out1) -> m/1
  Gain/1 -> Controlled Current Source/1
  connections:
  Voltage Measurement1/LConn1 -- Series RLC Branch/LConn1 -- a/RConn1 -- Controlled Current Source/RConn1
  Voltage Measurement1/LConn2 -- Series RLC Branch/RConn1 -- b/RConn1 -- Controlled Current Source/LConn1

== system IEEE34_SPSload/SM_IEEE34/DL_832-858/Load B ==
  Controlled Current Source : spsControlledCurrentSourceLib/Controlled Current Source  Initialize=on  Source_Type=AC  Amplitude=0  Phase=0  Frequency=0  Measurements=None
  Gain : Gain  Gain=-1
  Measurement list : Subsystem
  PQ : Ground
  Series RLC Branch : spsSeriesRLCBranchLib/Series RLC Branch  LConnTagsString=__new0  RConnTagsString=__new0  BranchType=R  Resistance=1e8  Inductance=1e-3  SetiL0=off  InitialCurrent=0  Capacitance=1e-6  Setx0=off  InitialVoltage=0  Measurements=None
  Voltage Measurement1 : spsVoltageMeasurementLib/Voltage Measurement  PhasorSimulation=off  OutputType=Complex  PSBequivalent=0
  model : Subsystem
  a : PMIOPort  Tag=PMCPort  Side=Left
  b : PMIOPort  Tag=PMCPort  Port=2  Side=Left
  m : Outport  InitialOutput=[0,0,0]  VectorParamsAs1DForOutWhenUnconnected=off
  wires:
  Gain/1 -> Controlled Current Source/1
  Measurement list/1(Out1) -> m/1
  model/1(i) -> Gain/1
  Voltage Measurement1/1 -> model/1(v)
  PQ/1 -> model/2(PQ)
  model/2(m) -> Measurement list/1(In1)
  connections:
  Controlled Current Source/LConn1 -- b/RConn1 -- Series RLC Branch/RConn1 -- Voltage Measurement1/LConn2
  Controlled Current Source/RConn1 -- a/RConn1 -- Series RLC Branch/LConn1 -- Voltage Measurement1/LConn1

== system IEEE34_SPSload/SM_IEEE34/DL_832-858/Load C ==
  Controlled Current Source : spsControlledCurrentSourceLib/Controlled Current Source  Initialize=on  Source_Type=AC  Amplitude=0  Phase=0  Frequency=0  Measurements=None
  Gain : Gain  Gain=-1
  Measurement list : Subsystem
  PQ : Ground
  Series RLC Branch : spsSeriesRLCBranchLib/Series RLC Branch  LConnTagsString=__new0  RConnTagsString=__new0  BranchType=R  Resistance=1e8  Inductance=1e-3  SetiL0=off  InitialCurrent=0  Capacitance=1e-6  Setx0=off  InitialVoltage=0  Measurements=None
  Voltage Measurement1 : spsVoltageMeasurementLib/Voltage Measurement  PhasorSimulation=off  OutputType=Complex  PSBequivalent=0
  model : Subsystem
  a : PMIOPort  Tag=PMCPort  Side=Left
  b : PMIOPort  Tag=PMCPort  Port=2  Side=Left
  m : Outport  InitialOutput=[0,0,0]  VectorParamsAs1DForOutWhenUnconnected=off
  wires:
  model/2(m) -> Measurement list/1(In1)
  PQ/1 -> model/2(PQ)
  Voltage Measurement1/1 -> model/1(v)
  model/1(i) -> Gain/1
  Measurement list/1(Out1) -> m/1
  Gain/1 -> Controlled Current Source/1
  connections:
  Voltage Measurement1/LConn1 -- Series RLC Branch/LConn1 -- a/RConn1 -- Controlled Current Source/RConn1
  Voltage Measurement1/LConn2 -- Series RLC Branch/RConn1 -- b/RConn1 -- Controlled Current Source/LConn1

== system IEEE34_SPSload/SM_IEEE34/DL_834-1/Load B ==
  Controlled Current Source : spsControlledCurrentSourceLib/Controlled Current Source  Initialize=on  Source_Type=AC  Amplitude=0  Phase=0  Frequency=0  Measurements=None
  Gain : Gain  Gain=-1
  Measurement list : Subsystem
  PQ : Ground
  Series RLC Branch : spsSeriesRLCBranchLib/Series RLC Branch  LConnTagsString=__new0  RConnTagsString=__new0  BranchType=R  Resistance=1e8  Inductance=1e-3  SetiL0=off  InitialCurrent=0  Capacitance=1e-6  Setx0=off  InitialVoltage=0  Measurements=None
  Voltage Measurement1 : spsVoltageMeasurementLib/Voltage Measurement  PhasorSimulation=off  OutputType=Complex  PSBequivalent=0
  model : Subsystem
  a : PMIOPort  Tag=PMCPort  Side=Left
  b : PMIOPort  Tag=PMCPort  Port=2  Side=Left
  m : Outport  InitialOutput=[0,0,0]  VectorParamsAs1DForOutWhenUnconnected=off
  wires:
  Gain/1 -> Controlled Current Source/1
  Measurement list/1(Out1) -> m/1
  model/1(i) -> Gain/1
  Voltage Measurement1/1 -> model/1(v)
  PQ/1 -> model/2(PQ)
  model/2(m) -> Measurement list/1(In1)
  connections:
  Controlled Current Source/LConn1 -- b/RConn1 -- Series RLC Branch/RConn1 -- Voltage Measurement1/LConn2
  Controlled Current Source/RConn1 -- a/RConn1 -- Series RLC Branch/LConn1 -- Voltage Measurement1/LConn1

== system IEEE34_SPSload/SM_IEEE34/DL_834-1/Load B1 ==
  Controlled Current Source : spsControlledCurrentSourceLib/Controlled Current Source  Initialize=on  Source_Type=AC  Amplitude=0  Phase=0  Frequency=0  Measurements=None
  Gain : Gain  Gain=-1
  Measurement list : Subsystem
  PQ : Ground
  Series RLC Branch : spsSeriesRLCBranchLib/Series RLC Branch  LConnTagsString=__new0  RConnTagsString=__new0  BranchType=R  Resistance=1e8  Inductance=1e-3  SetiL0=off  InitialCurrent=0  Capacitance=1e-6  Setx0=off  InitialVoltage=0  Measurements=None
  Voltage Measurement1 : spsVoltageMeasurementLib/Voltage Measurement  PhasorSimulation=off  OutputType=Complex  PSBequivalent=0
  model : Subsystem
  a : PMIOPort  Tag=PMCPort  Side=Left
  b : PMIOPort  Tag=PMCPort  Port=2  Side=Left
  m : Outport  InitialOutput=[0,0,0]  VectorParamsAs1DForOutWhenUnconnected=off
  wires:
  Gain/1 -> Controlled Current Source/1
  Measurement list/1(Out1) -> m/1
  model/1(i) -> Gain/1
  Voltage Measurement1/1 -> model/1(v)
  PQ/1 -> model/2(PQ)
  model/2(m) -> Measurement list/1(In1)
  connections:
  Controlled Current Source/LConn1 -- b/RConn1 -- Series RLC Branch/RConn1 -- Voltage Measurement1/LConn2
  Controlled Current Source/RConn1 -- a/RConn1 -- Series RLC Branch/LConn1 -- Voltage Measurement1/LConn1

== system IEEE34_SPSload/SM_IEEE34/DL_834-1/Load B2 ==
  Controlled Current Source : spsControlledCurrentSourceLib/Controlled Current Source  Initialize=on  Source_Type=AC  Amplitude=0  Phase=0  Frequency=0  Measurements=None
  Gain : Gain  Gain=-1
  Measurement list : Subsystem
  PQ : Ground
  Series RLC Branch : spsSeriesRLCBranchLib/Series RLC Branch  LConnTagsString=__new0  RConnTagsString=__new0  BranchType=R  Resistance=1e8  Inductance=1e-3  SetiL0=off  InitialCurrent=0  Capacitance=1e-6  Setx0=off  InitialVoltage=0  Measurements=None
  Voltage Measurement1 : spsVoltageMeasurementLib/Voltage Measurement  PhasorSimulation=off  OutputType=Complex  PSBequivalent=0
  model : Subsystem
  a : PMIOPort  Tag=PMCPort  Side=Left
  b : PMIOPort  Tag=PMCPort  Port=2  Side=Left
  m : Outport  InitialOutput=[0,0,0]  VectorParamsAs1DForOutWhenUnconnected=off
  wires:
  Gain/1 -> Controlled Current Source/1
  Measurement list/1(Out1) -> m/1
  model/1(i) -> Gain/1
  Voltage Measurement1/1 -> model/1(v)
  PQ/1 -> model/2(PQ)
  model/2(m) -> Measurement list/1(In1)
  connections:
  Controlled Current Source/LConn1 -- b/RConn1 -- Series RLC Branch/RConn1 -- Voltage Measurement1/LConn2
  Controlled Current Source/RConn1 -- a/RConn1 -- Series RLC Branch/LConn1 -- Voltage Measurement1/LConn1

== system IEEE34_SPSload/SM_IEEE34/DL_834-860/Load B ==
  Controlled Current Source : spsControlledCurrentSourceLib/Controlled Current Source  Initialize=on  Source_Type=AC  Amplitude=0  Phase=0  Frequency=0  Measurements=None
  Gain : Gain  Gain=-1
  Measurement list : Subsystem
  PQ : Ground
  Series RLC Branch : spsSeriesRLCBranchLib/Series RLC Branch  LConnTagsString=__new0  RConnTagsString=__new0  BranchType=R  Resistance=1e8  Inductance=1e-3  SetiL0=off  InitialCurrent=0  Capacitance=1e-6  Setx0=off  InitialVoltage=0  Measurements=None
  Voltage Measurement1 : spsVoltageMeasurementLib/Voltage Measurement  PhasorSimulation=off  OutputType=Complex  PSBequivalent=0
  model : Subsystem
  a : PMIOPort  Tag=PMCPort  Side=Left
  b : PMIOPort  Tag=PMCPort  Port=2  Side=Left
  m : Outport  InitialOutput=[0,0,0]  VectorParamsAs1DForOutWhenUnconnected=off
  wires:
  model/2(m) -> Measurement list/1(In1)
  PQ/1 -> model/2(PQ)
  Voltage Measurement1/1 -> model/1(v)
  model/1(i) -> Gain/1
  Measurement list/1(Out1) -> m/1
  Gain/1 -> Controlled Current Source/1
  connections:
  Voltage Measurement1/LConn1 -- Series RLC Branch/LConn1 -- a/RConn1 -- Controlled Current Source/RConn1
  Voltage Measurement1/LConn2 -- Series RLC Branch/RConn1 -- b/RConn1 -- Controlled Current Source/LConn1

== system IEEE34_SPSload/SM_IEEE34/DL_834-860/Load B1 ==
  Controlled Current Source : spsControlledCurrentSourceLib/Controlled Current Source  Initialize=on  Source_Type=AC  Amplitude=0  Phase=0  Frequency=0  Measurements=None
  Gain : Gain  Gain=-1
  Measurement list : Subsystem
  PQ : Ground
  Series RLC Branch : spsSeriesRLCBranchLib/Series RLC Branch  LConnTagsString=__new0  RConnTagsString=__new0  BranchType=R  Resistance=1e8  Inductance=1e-3  SetiL0=off  InitialCurrent=0  Capacitance=1e-6  Setx0=off  InitialVoltage=0  Measurements=None
  Voltage Measurement1 : spsVoltageMeasurementLib/Voltage Measurement  PhasorSimulation=off  OutputType=Complex  PSBequivalent=0
  model : Subsystem
  a : PMIOPort  Tag=PMCPort  Side=Left
  b : PMIOPort  Tag=PMCPort  Port=2  Side=Left
  m : Outport  InitialOutput=[0,0,0]  VectorParamsAs1DForOutWhenUnconnected=off
  wires:
  model/2(m) -> Measurement list/1(In1)
  PQ/1 -> model/2(PQ)
  Voltage Measurement1/1 -> model/1(v)
  model/1(i) -> Gain/1
  Measurement list/1(Out1) -> m/1
  Gain/1 -> Controlled Current Source/1
  connections:
  Voltage Measurement1/LConn1 -- Series RLC Branch/LConn1 -- a/RConn1 -- Controlled Current Source/RConn1
  Voltage Measurement1/LConn2 -- Series RLC Branch/RConn1 -- b/RConn1 -- Controlled Current Source/LConn1

== system IEEE34_SPSload/SM_IEEE34/DL_834-860/Load B2 ==
  Controlled Current Source : spsControlledCurrentSourceLib/Controlled Current Source  Initialize=on  Source_Type=AC  Amplitude=0  Phase=0  Frequency=0  Measurements=None
  Gain : Gain  Gain=-1
  Measurement list : Subsystem
  PQ : Ground
  Series RLC Branch : spsSeriesRLCBranchLib/Series RLC Branch  LConnTagsString=__new0  RConnTagsString=__new0  BranchType=R  Resistance=1e8  Inductance=1e-3  SetiL0=off  InitialCurrent=0  Capacitance=1e-6  Setx0=off  InitialVoltage=0  Measurements=None
  Voltage Measurement1 : spsVoltageMeasurementLib/Voltage Measurement  PhasorSimulation=off  OutputType=Complex  PSBequivalent=0
  model : Subsystem
  a : PMIOPort  Tag=PMCPort  Side=Left
  b : PMIOPort  Tag=PMCPort  Port=2  Side=Left
  m : Outport  InitialOutput=[0,0,0]  VectorParamsAs1DForOutWhenUnconnected=off
  wires:
  model/2(m) -> Measurement list/1(In1)
  PQ/1 -> model/2(PQ)
  Voltage Measurement1/1 -> model/1(v)
  model/1(i) -> Gain/1
  Measurement list/1(Out1) -> m/1
  Gain/1 -> Controlled Current Source/1
  connections:
  Voltage Measurement1/LConn1 -- Series RLC Branch/LConn1 -- a/RConn1 -- Controlled Current Source/RConn1
  Voltage Measurement1/LConn2 -- Series RLC Branch/RConn1 -- b/RConn1 -- Controlled Current Source/LConn1

== system IEEE34_SPSload/SM_IEEE34/DL_842-1/Load B ==
  Controlled Current Source : spsControlledCurrentSourceLib/Controlled Current Source  Initialize=on  Source_Type=AC  Amplitude=0  Phase=0  Frequency=0  Measurements=None
  Gain : Gain  Gain=-1
  Measurement list : Subsystem
  PQ : Ground
  Series RLC Branch : spsSeriesRLCBranchLib/Series RLC Branch  LConnTagsString=__new0  RConnTagsString=__new0  BranchType=R  Resistance=1e8  Inductance=1e-3  SetiL0=off  InitialCurrent=0  Capacitance=1e-6  Setx0=off  InitialVoltage=0  Measurements=None
  Voltage Measurement1 : spsVoltageMeasurementLib/Voltage Measurement  PhasorSimulation=off  OutputType=Complex  PSBequivalent=0
  model : Subsystem
  a : PMIOPort  Tag=PMCPort  Side=Left
  b : PMIOPort  Tag=PMCPort  Port=2  Side=Left
  m : Outport  InitialOutput=[0,0,0]  VectorParamsAs1DForOutWhenUnconnected=off
  wires:
  Gain/1 -> Controlled Current Source/1
  Measurement list/1(Out1) -> m/1
  model/1(i) -> Gain/1
  Voltage Measurement1/1 -> model/1(v)
  PQ/1 -> model/2(PQ)
  model/2(m) -> Measurement list/1(In1)
  connections:
  Controlled Current Source/LConn1 -- b/RConn1 -- Series RLC Branch/RConn1 -- Voltage Measurement1/LConn2
  Controlled Current Source/RConn1 -- a/RConn1 -- Series RLC Branch/LConn1 -- Voltage Measurement1/LConn1
